simulink model "ondinhbangbang"  (R2022a)
settings: Solver=VariableStepAuto  StartTime=0.0  StopTime=10.0  RelTol=1e-3
libraries: arduinolib x2
settings Model: Creator=TUAN  LastModifiedBy=TUAN

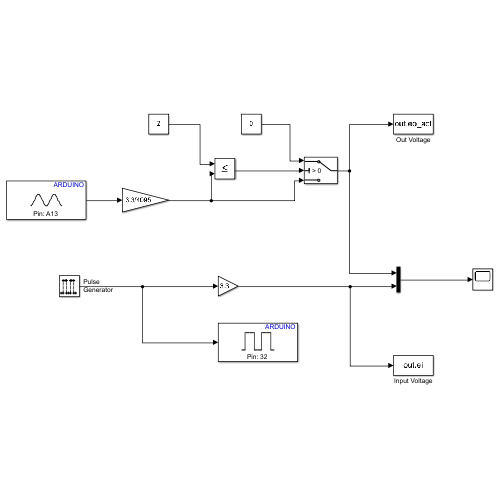
[thumbnail: Simulink's stored preview of the top-level diagram]
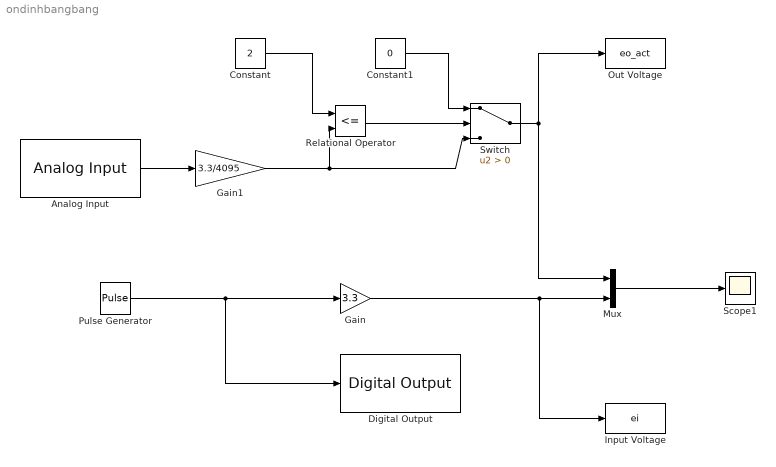
== system ondinhbangbang ==
  Analog Input : arduinolib/Analog Input  pinNumber=13  ReadResultsOnly=off  ConversionTriggerSource=Software  ExternalTriggerType=uint32( 0 )  OutputDataType=uint16  EnableConversionCompleteNotify=off  EnableOuputStatus=off  SampleTime=0.001  blockPlatform=arduino
  Constant : Constant  Value=2
  Constant1 : Constant  Value=0
  Digital Output : arduinolib/Digital Output  pinNumber=32  Direction=output  blockPlatform=arduino
  Gain : Gain  Gain=3.3
  Gain1 : Gain  Gain=3.3/4095  OutDataTypeStr=double
  Input Voltage : ToWorkspace  VariableName=ei  SampleTime=-1
  Mux : Mux  Inputs=2
  Out Voltage : ToWorkspace  VariableName=eo_act  SampleTime=-1
      settings: Save2DSignal=2-D array (concatenate along first dimension)
  Pulse Generator : DiscretePulseGenerator  Period=100  PulseWidth=50  SampleTime=0.1
  Relational Operator : RelationalOperator  Operator=<=  OutDataTypeStr=boolean  RndMeth=Simplest  InputSameDT=off
  Scope1 : Scope
  Switch : Switch  Criteria=u2 > Threshold  SaturateOnIntegerOverflow=off  InputSameDT=off
  wires:
  Gain/1 -> Input Voltage/1, Mux/2
  Mux/1 -> Scope1/1
  Constant/1 -> Relational Operator/1
  Constant1/1 -> Switch/1
  Gain1/1 -> Relational Operator/2, Switch/3
  Pulse Generator/1 -> Digital Output/1, Gain/1
  Analog Input/1 -> Gain1/1
  Relational Operator/1 -> Switch/2
  Switch/1 -> Mux/1, Out Voltage/1
